simulink model "drone_simulation_3D_step_response"  (R2022b)
settings: Solver=FixedStepAuto  StartTime=0.0  StopTime=1  FixedStep=0.001  RelTol=1e-3
model workspace (MAT data in the model file):
  amplitude = 0.05
settings Model: Creator=andre  LastModifiedBy=UNI

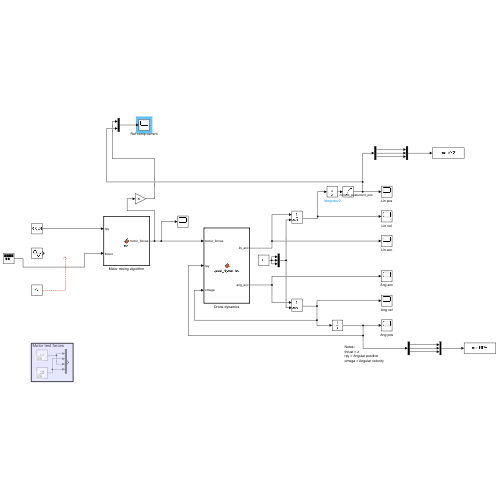
[thumbnail: Simulink's stored preview of the top-level diagram]
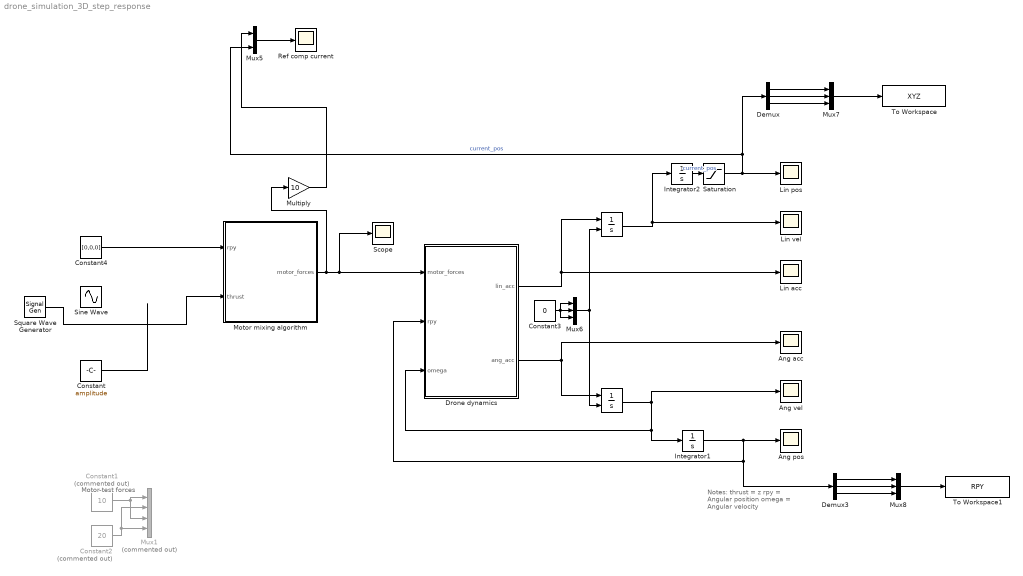
== system drone_simulation_3D_step_response ==
  note: Notes:
      | thrust = z
      | rpy = Angular position
      | omega = Angular velocity
  note: Motor test forces
  " " : Integrator  InitialConditionSource=external  InitialCondition=[0;0;0]
  "  " : Integrator  InitialConditionSource=external  InitialCondition=[0;0;0]
  Ang acc : Scope
  Ang pos : Scope
  Ang vel : Scope
  Constant : Constant  Value=amplitude
  Constant1 : Constant  Commented=on  Value=10
  Constant2 : Constant  Commented=on  Value=20
  Constant3 : Constant  Value=0
  Constant4 : Constant  Value=[0,0,0]
  Demux : Demux  Outputs=3
  Demux3 : Demux  Outputs=3
  Drone dynamics : MATLAB Function  TreatAsAtomicUnit=on
  Integrator1 : Integrator
  Integrator2 : Integrator
  Lin acc : Scope
  Lin pos : Scope
  Lin vel : Scope
  Motor mixing algorithm : MATLAB Function  TreatAsAtomicUnit=on
  Multiply : Gain  Gain=10
  Mux1 : Mux  Commented=on
  Mux5 : Mux  Inputs=2
  Mux6 : Mux  Inputs=3
  Mux7 : Mux  Inputs=3
  Mux8 : Mux  Inputs=3
  Ref comp current : Scope
  Saturation : Saturate  UpperLimit=inf  LowerLimit=0
  Scope : Scope
  Sine Wave : Sin  SampleTime=0
  Square Wave Generator : SignalGenerator  WaveForm=square  Amplitude=-0.1  Units=rad/sec
  To Workspace : ToWorkspace  VariableName=XYZ  SampleTime=-1
  To Workspace1 : ToWorkspace  VariableName=RPY  SampleTime=-1
  wires:
  Drone dynamics/1(lin_acc) -> " "/1, Lin acc/1
  Drone dynamics/2(ang_acc) -> Ang acc/1, "  "/1
  "  "/1 -> Ang vel/1, Drone dynamics/3(omega), Integrator1/1
  Integrator1/1 -> Demux3/1, Drone dynamics/2(rpy), Ang pos/1
  " "/1 -> Integrator2/1, Lin vel/1
  Saturation/1 -> Demux/1, Mux5/2, Lin pos/1  "current_pos"
  Constant1/1 -> Mux1/3, Mux1/1
  Constant2/1 -> Mux1/4, Mux1/2
  Constant4/1 -> Motor mixing algorithm/1(rpy)
  Motor mixing algorithm/1(motor_forces) -> Multiply/1, Scope/1, Drone dynamics/1(motor_forces)
  Mux5/1 -> Ref comp current/1
  Constant3/1 -> Mux6/3, Mux6/1, Mux6/2
  Mux6/1 -> "  "/2, " "/2
  Demux/1 -> Mux7/1
  Demux/2 -> Mux7/2
  Demux/3 -> Mux7/3
  Mux7/1 -> To Workspace/1
  Demux3/2 -> Mux8/2
  Mux8/1 -> To Workspace1/1
  Demux3/1 -> Mux8/1
  Demux3/3 -> Mux8/3
  Integrator2/1 -> Saturation/1  "current_pos"
  Constant/1 -> ?
  Multiply/1 -> Mux5/1
  Square Wave Generator/1 -> Motor mixing algorithm/2(thrust)

== matlab function drone_simulation_3D_step_response/Motor mixing algorithm ==
  data: motor_forces output size=[1, 4]; rpy input size=[1, 3]; thrust input
function motor_forces = fcn(rpy, thrust)

% r = rpy(1);
% p = rpy(2);
% y = rpy(3);
% 
% motor_forces = ...
% [sum([r   p   y thrust]); ...
% sum([-r   p  -y thrust]);   ...
% sum([-r  -p   y thrust]);   ...
% sum([ r  -p  -y thrust])];

m1 = thrust + rpy(1) - rpy(2) - rpy(3);
m2 = thrust - rpy(1) - rpy(2) + rpy(3);
m3 = thrust - rpy(1) + rpy(2) - rpy(3);
m4 = thrust + rpy(1) + rpy(2) + rpy(3);
motor_forces = [m1, m2, m3, m4];

== matlab function drone_simulation_3D_step_response/Drone dynamics ==
  data: motor_forces input; lin_acc output; rpy input; ang_acc output; omega input
function [lin_acc, ang_acc] = quad_dynamics(motor_forces, rpy, omega)



%% Define constants
rotor_dist = 0.04; %m
body_mass = 0.02989; %kg
g_constant = [0;0;-9.82]; %Nm/s^2




% Vectors from CoM to motors
% We create a X-configured drone
rotor_angle = pi/4;
s1 = [cos(rotor_angle); sin(rotor_angle); 0] * rotor_dist;
s2 = [cos(rotor_angle); -sin(rotor_angle); 0] * rotor_dist;
s3 = [-cos(rotor_angle); -sin(rotor_angle); 0] * rotor_dist;
s4 = [-cos(rotor_angle); sin(rotor_angle); 0] * rotor_dist;
s_vectors = [s1 s2 s3 s4];

% Local motor force vectors
m1_vec = [0;0;motor_forces(1)];
m2_vec = [0;0;motor_forces(2)];
m3_vec = [0;0;motor_forces(3)];
m4_vec = [0;0;motor_forces(4)];
local_motor_forces = [m1_vec m2_vec m3_vec m4_vec];
    



%change the minuses if it rotates in the wrong direction, they are just
%random now
tau2m1 = [0;0;-thrust2torque(motor_forces(1))];
tau2m2 = [0;0; thrust2torque(motor_forces(2))];
tau2m3 = [0;0;-thrust2torque(motor_forces(3))];
tau2m4 = [0;0; thrust2torque(motor_forces(4))];
local_motor_torques = [tau2m1 tau2m2 tau2m3 tau2m4];

% Local inertia tensor
I_local = [1.132869584e-05 0 0; 0 1.132869584e-05 0; 0 0 2.028869584e-05];



%% Calculate drone components

% Rotation matrix
%R = rpy2r(rpy(1), rpy(2), rpy(3));
R = rotx(rpy(1)) * roty(rpy(2)) * rotz(rpy(3));

% Global inertia tensor
I_global = (R * I_local) * transpose(R);


%% Equation of motion

% Total force
total_force = R * sum(local_motor_forces,2) + (body_mass * g_constant);

% Total moment
total_moment = R * (sum(cross(s_vectors,local_motor_forces),2)+sum(local_motor_torques,2));

%% Linear and angular acceleration
a = total_force/body_mass;
lin_acc = [a(1) a(2) a(3)];

alpha = inv(I_global) * (total_moment - cross(omega,(I_global * omega)));
ang_acc = [alpha(1) alpha(2) alpha(3)];
% omega = angular velocity
% alpha = angular acceleration
end
